simulink model "ModeInputHandle"  (R2018b)
settings: Solver=FixedStepDiscrete  StartTime=0.0  StopTime=10.0  FixedStep=0.01  RelTol=1e-3
undefined symbols (not defined in the file or in its folder): c, CmprtMdHMIReqExt2Tp1, CmprtMdHMIReqExtTp1, CmprtMdHMIReqTp1, d, e, EZESwReq1, f, g, IfVeSMSeStNumConfig, j, KeSMSuButtonLongPressedThrshldTm_Val, KeSMSuFoldType_Val, KeSMSwSeatSMSSeatMdTrigGapTimer_Val, KeSMSwSeatTrigWaitTimer_Val, KeSMSwSRSActiveValidTm_Val, LckUlckActvtFunc1, LstLckFunc1, LugSelectSw1, MdReqTp1, PowerMode1, SeatOccupiedSts1, SRSMode1, StPassCmprtMdCtrl_Md10_VCUConfig_Val, StPassCmprtMdCtrl_Md11_VCUConfig_Val, StPassCmprtMdCtrl_Md12_VCUConfig_Val, StPassCmprtMdCtrl_Md13_VCUConfig_Val, StPassCmprtMdCtrl_Md1_VCUConfig_Val, StPassCmprtMdCtrl_Md27_VCUConfig_Val, StPassCmprtMdCtrl_Md28_VCUConfig_Val, StPassCmprtMdCtrl_Md29_VCUConfig_Val, StPassCmprtMdCtrl_Md2_VCUConfig_Val, StPassCmprtMdCtrl_Md30_VCUConfig_Val, StPassCmprtMdCtrl_Md31_VCUConfig_Val, StPassCmprtMdCtrl_Md32_VCUConfig_Val, StPassCmprtMdCtrl_Md3_VCUConfig_Val, StPassCmprtMdCtrl_Md53_VCUConfig_Val, StPassCmprtMdCtrl_Md56_VCUConfig_Val, StPassCmprtMdCtrl_Md57_VCUConfig_Val, StPassCmprtMdCtrl_Md58_VCUConfig_Val, StPassCmprtMdCtrl_Md61_VCUConfig_Val, StPassCmprtMdCtrl_Md62_VCUConfig_Val, StPassCmprtMdCtrl_Md8_VCUConfig_Val, StPassCmprtMdCtrl_Md9_VCUConfig_Val, StSrv_StMd10_Config_Val, StSrv_StMd11_Config_Val, StSrv_StMd12_Config_Val, StSrv_StMd13_Config_Val, StSrv_StMd1_Config_Val, StSrv_StMd27_Config_Val, StSrv_StMd28_Config_Val, StSrv_StMd29_Config_Val, StSrv_StMd2_Config_Val, StSrv_StMd30_Config_Val, StSrv_StMd31_Config_Val, StSrv_StMd32_Config_Val, StSrv_StMd3_Config_Val, StSrv_StMd8_Config_Val, StSrv_StMd9_Config_Val, VehMovState1
libraries: MSMLib x91
(part 4 of 9)

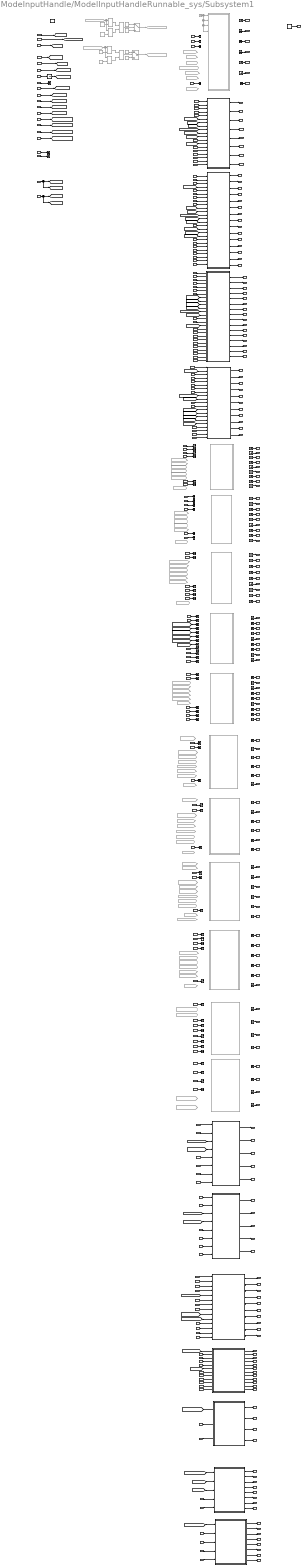
== system ModeInputHandle/ModelInputHandleRunnable_sys/Subsystem1 ==
  note: 2022-02-17:CR202175：修改需求506/548/551/552，新增需求712，完善座椅模式的打断策略。
      | 2023-08-01:新增mode21~26控制接口，REQ_MSM_772/773/774/775//781/784
      | 2024-01-25:对应CT698686:增加KeSMSwSeatTrigWaitTimer，修复休眠情况下无法自动迎宾的问题
  note: //init=[0 1 2 4 3 0 0 0 0 0 0]
  AcsMdExtMdHMI2LRclReq : Inport
  AcsMdExtMdHMI2RRclReq : Inport  Port=2
  AcsMdExtSwLtRclReq : Inport  Port=3
  AcsMdExtSwLtRclReqV : Inport  Port=4
  AcsMdExtSwRtRclReq : Inport  Port=5
  AcsMdExtSwRtRclReqV : Inport  Port=6
  StPassAcsMdExtReq : Inport  Port=7
  SRSCnfmSwReq_67_2 : Inport  Port=8
  StPassCmprtMdHMIReq : Inport  Port=9
  modeAdjustReqDelay : Inport  Port=10
  AcsMdEtrySwRtRclReq : Inport  Port=11
  AcsMdEtrySwRtRclReqV : Inport  Port=12
  AcsEntry2LSwt : Inport  Port=13
  StPassAcsMdEtryReq : Inport  Port=14
  VipMdSwRtRclReq : Inport  Port=15
  VipMdSwRtRclReqV : Inport  Port=16
  Vip2LSwt : Inport  Port=17
  VIPMdHMI2LRclReq : Inport  Port=18
  VIPMdHMI2RRclReq : Inport  Port=19
  StPassVipMdLtReq : Inport  Port=20
  StPassVipMdRtReq : Inport  Port=21
  StSlctSwReq : Inport  Port=22
  StSlctSwReqV : Inport  Port=23
  LugMdSwRclReq : Inport  Port=24
  LugMdSwRclReqV : Inport  Port=25
  StPassLugMdLtReq : Inport  Port=26
  StPassLugMdRtReq : Inport  Port=27
  StPassRcvyMdLtReq : Inport  Port=28
  StPassRcvyMdRtReq : Inport  Port=29
  RcvySwRtReq : Inport  Port=30
  RcvySwRtReqV : Inport  Port=31
  Recovery2LSwt : Inport  Port=32
  RcvyMdHMI2LRclReq : Inport  Port=33
  RcvyMdHMI2RRclReq : Inport  Port=34
  RcvyMdLtAvl : Inport  Port=35
  RcvyMdRtAvl : Inport  Port=36
  ModeSrcTpLt : Inport  Port=37
  KeSMSwSRSActiveValidTm : Inport  Port=38
  KeSMSuButtonLongPressedThrshldTm : Inport  Port=39
  AcsMdExtAvl : Inport  Port=40
  AcsMdEntyAvl : Inport  Port=41
  VipMdLtAvl : Inport  Port=42
  VipMdRtAvl : Inport  Port=43
  LugMdLtAvl : Inport  Port=44
  LugMdRtAvl : Inport  Port=45
  RrRcvyMdSwRclReq : Inport  Port=46
  RrRcvyMdSwRclReqV : Inport  Port=47
  SRSMode : Inport  Port=48
  StPassCmprtMdHMIReqExt : Inport  Port=49
  AcsMdEntyHMI2LRclReq : Inport  Port=50
  AcsMdEntyHMI2RRclReq : Inport  Port=51
  VIPAll2LHMIRclReq : Inport  Port=52
  VIPAll2RHMIRclReq : Inport  Port=53
  Lug2LHMIRclReq : Inport  Port=54
  Lug2RHMIRclReq : Inport  Port=55
  LugAll2LHMIRclReq : Inport  Port=56
  LugAll2RHMIRclReq : Inport  Port=57
  StPassVipAllReq : Inport  Port=58
  StPassLugAllReq : Inport  Port=59
  StPassIntimacyLtMdReq : Inport  Port=60
  StPassIntimacyRtMdReq : Inport  Port=61
  IntimacyLMdHMI2LRclReq : Inport  Port=62
  IntimacyRMdHMI2RRclReq : Inport  Port=63
  IntimacyLMdAvl : Inport  Port=64
  IntimacyRMdAvl : Inport  Port=65
  StPassFamilyMdLtReq : Inport  Port=66
  FamilyMdHMI2LRclReq : Inport  Port=67
  FamilyMdHMI2RRclReq : Inport  Port=68
  FamilyMdLtAvl : Inport  Port=69
  PassFamilyMdRtReq : Inport  Port=70
  FamilyMdRtAvl : Inport  Port=71
  PassLyingMdLtReq : Inport  Port=72
  PassLyingMdRtReq : Inport  Port=73
  LyingMdHMI2LRclReq : Inport  Port=74
  LyingMdHMI2RRclReq : Inport  Port=75
  LyingMdLtAvl : Inport  Port=76
  LyingMdRtAvl : Inport  Port=77
  AcsEntrySwValid : Inport  Port=78
  VipRcvySwValid : Inport  Port=79
  PassLgrstOpenLtMdReq : Inport  Port=80
  PassLgrstCloseLtMdReq : Inport  Port=81
  LgrstOpenLtMdAvl : Inport  Port=82
  LgrstCloseLtMdAvl : Inport  Port=83
  LgrstOpenLtMdHMI2LRclReq : Inport  Port=84
  LgrstCloseLtMdHMI2LRclReq : Inport  Port=85
  PassLgrstOpenRtMdReq : Inport  Port=86
  PassLgrstCloseRtMdReq : Inport  Port=87
  LgrstOpenRtMdAvl : Inport  Port=88
  LgrstCloseRtMdAvl : Inport  Port=89
  LgrstOpenRtMdHMI2RRclReq : Inport  Port=90
  LgrstCloseRtMdHMI2RRclReq : Inport  Port=91
  SRSSlctSwReq : Inport  Port=92
  AcsEntry4s2LAvl : Inport  Port=93
  EZE4SSwReq : Inport  Port=94
  HMIMode21RclReq_2L : Inport  Port=95
  PassAcsEntry4s2LReq : Inport  Port=96
  AcsExit4s2LAvl : Inport  Port=97
  HMIMode22RclReq_2L : Inport  Port=98
  PassAcsExit4s2LReq : Inport  Port=99
  AcsEntry4s2RAvl : Inport  Port=100
  HMIMode23RclReq_2R : Inport  Port=101
  PassAcsEntry4s2RReq : Inport  Port=102
  AcsExit4s2RAvl : Inport  Port=103
  AcsMdExt4SSwRtRclReq : Inport  Port=104
  AcsMdExt4SSwRtRclReqV : Inport  Port=105
  HMIMode24RclReq_2R : Inport  Port=106
  PassAcsExit4s2RReq : Inport  Port=107
  LckUlckActvtFunc : Inport  Port=108
  NotSecRowLeSeaOccStat : Inport  Port=109
  NotSecRowRtSeaOccStat : Inport  Port=110
  SysPwrMd : Inport  Port=111
  SysPwrMdV : Inport  Port=112
  VehMovState : Inport  Port=113
  AcsEntryAll4sFwdAvl : Inport  Port=114
  LstLckFunc : Inport  Port=115
  LstLckChange : Inport  Port=116
  RLDoorAjarSwAct : Inport  Port=117
  RRDoorAjarSwAct : Inport  Port=118
  KeSMSwSeatSMSSeatMdTrigGapTimer : Inport  Port=119
  AcsEntryAll4sBwdAvl : Inport  Port=120
  IfVeSMSeStNumConfig_Val_read : Inport  Port=121
  KeSMSwSeatTrigWaitTimer : Inport  Port=122
  PasReclinerAvl : Inport  Port=123
  PassStFldDnMovSwAct : Inport  Port=124
  PassStFldDnMovSwActV : Inport  Port=125
  PassStFldUpMovSwAct : Inport  Port=126
  PassStFldUpMovSwActV : Inport  Port=127
  StPassPasReclinerEntryReq : Inport  Port=128
  StPassPasReclinerExitReq : Inport  Port=129
  ThdRLtStExpdSwReq : Inport  Port=130
  ThdRLtStExpdSwReqV : Inport  Port=131
  ThdRRtStExpdSwReq : Inport  Port=132
  ThdRRtStExpdSwReqV : Inport  Port=133
  KeSMSuFoldType : Inport  Port=134
  unfold3LAvl : Inport  Port=135
  unfold3RAvl : Inport  Port=136
  VipLtOutMdAvl : Inport  Port=137
  VipRtOutMdAvl : Inport  Port=138
  StPassVIPLtOutReq : Inport  Port=139
  StPassVIPRtOutReq : Inport  Port=140
  StPassVIPAllOutReq : Inport  Port=141
  PasReclinerExitAvl : Inport  Port=142
  StPassCmprtMdHMIReqExt2 : Inport  Port=143
  StPassUnfold3LReq : Inport  Port=144
  Big4SeatAvl : Inport  Port=145
  M61WholeVehMemAvl : Inport  Port=146
  M62WholeVehMemAvl : Inport  Port=147
  StPassCmprtMdCtrl_Md1_VCUConfig : Inport  Port=148
  StPassCmprtMdCtrl_Md10_VCUConfig : Inport  Port=149
  StPassCmprtMdCtrl_Md11_VCUConfig : Inport  Port=150
  StPassCmprtMdCtrl_Md12_VCUConfig : Inport  Port=151
  StPassCmprtMdCtrl_Md13_VCUConfig : Inport  Port=152
  StPassCmprtMdCtrl_Md2_VCUConfig : Inport  Port=153
  StPassCmprtMdCtrl_Md27_VCUConfig : Inport  Port=154
  StPassCmprtMdCtrl_Md28_VCUConfig : Inport  Port=155
  StPassCmprtMdCtrl_Md29_VCUConfig : Inport  Port=156
  StPassCmprtMdCtrl_Md3_VCUConfig : Inport  Port=157
  StPassCmprtMdCtrl_Md30_VCUConfig : Inport  Port=158
  StPassCmprtMdCtrl_Md31_VCUConfig : Inport  Port=159
  StPassCmprtMdCtrl_Md32_VCUConfig : Inport  Port=160
  StPassCmprtMdCtrl_Md53_VCUConfig : Inport  Port=161
  StPassCmprtMdCtrl_Md56_VCUConfig : Inport  Port=162
  StPassCmprtMdCtrl_Md57_VCUConfig : Inport  Port=163
  StPassCmprtMdCtrl_Md58_VCUConfig : Inport  Port=164
  StPassCmprtMdCtrl_Md61_VCUConfig : Inport  Port=165
  StPassCmprtMdCtrl_Md62_VCUConfig : Inport  Port=166
  StPassCmprtMdCtrl_Md8_VCUConfig : Inport  Port=167
  StPassCmprtMdCtrl_Md9_VCUConfig : Inport  Port=168
  StSrv_StMd1_Config : Inport  Port=169
  StSrv_StMd10_Config : Inport  Port=170
  StSrv_StMd11_Config : Inport  Port=171
  StSrv_StMd12_Config : Inport  Port=172
  StSrv_StMd13_Config : Inport  Port=173
  StSrv_StMd2_Config : Inport  Port=174
  StSrv_StMd27_Config : Inport  Port=175
  StSrv_StMd28_Config : Inport  Port=176
  StSrv_StMd29_Config : Inport  Port=177
  StSrv_StMd3_Config : Inport  Port=178
  StSrv_StMd30_Config : Inport  Port=179
  StSrv_StMd31_Config : Inport  Port=180
  StSrv_StMd32_Config : Inport  Port=181
  StSrv_StMd8_Config : Inport  Port=182
  StSrv_StMd9_Config : Inport  Port=183
  AND2 : Logic  Commented=on  Operator=OR  AllPortsSameDT=off  OutDataTypeStr=boolean
  AND3 : Logic  Commented=on  Operator=OR  AllPortsSameDT=off  OutDataTypeStr=boolean
  AcsEntry4s2LMdReq : Subsystem  Commented=on
  "AcsEntry4s2RMdReq " : Subsystem  Commented=on
  AcsEntryAll4sBwdMdReq : Subsystem  Commented=on
  AcsEntryAll4sFwdMdReq : Subsystem  Commented=on
  AcsEntryMdReq : Subsystem
  AcsExit4s2LMdReq : Subsystem  Commented=on
  AcsExit4s2RMdReq : Subsystem  Commented=on
  AcsExtMdReq : Subsystem  Commented=on
  Big4SeatMdReq : Subsystem
  Constant : Constant  Commented=on  Value=IfVeSMSeStNumConfig.SeatNum7Config  OutDataTypeStr=Enum: IfVeSMSeStNumConfig
  Constant1 : Constant  Commented=on  Value=IfVeSMSeStNumConfig.SeatNum6Config  OutDataTypeStr=Enum: IfVeSMSeStNumConfig
  Constant2 : Constant  Commented=on  OutDataTypeStr=boolean
  Constant3 : Constant  Commented=on  Value=0  OutDataTypeStr=boolean
  Constant5 : Constant  Commented=on  Value=IfVeSMSeStNumConfig.SeatNum4Config  OutDataTypeStr=Enum: IfVeSMSeStNumConfig
  Constant6 : Constant  Commented=on  Value=IfVeSMSeStNumConfig.SeatNum4PConfig  OutDataTypeStr=Enum: IfVeSMSeStNumConfig
  Constant7 : Constant  Commented=on  OutDataTypeStr=boolean
  Constant8 : Constant  Commented=on  Value=0  OutDataTypeStr=boolean
  Data Store Memory : DataStoreMemory  DataStoreName=MdSWIntSrc_Val  ReadBeforeWriteMsg=warning  WriteAfterWriteMsg=warning  WriteAfterReadMsg=warning  ShowAdditionalParam=off  OutDataTypeStr=uint16
  Data Store Read : DataStoreRead  DataStoreName=MdSWIntSrc_Val
  Equal{,1..3} (4 alike) : RelationalOperator  Commented=on  Operator===  OutDataTypeStr=boolean  RndMeth=Simplest
  "ExVIPMdReq " : Subsystem
  FamilyMdReq : Subsystem  Commented=on
  From100 : From  Commented=on  GotoTag=NotSecRowRtSeaOccStat
  From{25,38,75,95,101} (5 alike) : From  Commented=on  GotoTag=buttonLongPressedThrshhldTm
  From102 : From  Commented=on  GotoTag=NotSecRowLeSeaOccStat
  From103 : From  Commented=on  GotoTag=NotSecRowRtSeaOccStat
  From105 : From  Commented=on  GotoTag=IfVeSMSeStNumConfig
  From106 : From  Commented=on  GotoTag=IfVeSMSeStNumConfig
  From107 : From  Commented=on  GotoTag=AcsEntry4s2RMdConfig
  From{20,35,61,68,84,91..92} (7 alike) : From  Commented=on  GotoTag=PassCmprtMdHMIReqExt
  From{5,21,40,52,57,62,85,90,98} (9 alike) : From  Commented=on  GotoTag=modeAdjustReqDelay
  From{22,36,53,58,63,69,86,93,230} (9 alike) : From  Commented=on  GotoTag=SRSSlctSwReq
  From{23,37,54,59,65,74,87,94,229} (9 alike) : From  Commented=on  GotoTag=SRSCnfmSwReq
  From{24,41,55,60,66,82,88,96,233} (9 alike) : From  Commented=on  GotoTag=SRSActiveValidTm
  From{26,30,42,71..73,83,89,97} (9 alike) : From  Commented=on  GotoTag=SRSMode
  From{27,46,56,64} (4 alike) : From  Commented=on  GotoTag=passCmprtMdHMIReq
  From28 : From  Commented=on  GotoTag=EZE4SSwReq
  From29 : From  Commented=on  GotoTag=EZE4SSwReq
  From45 : From  Commented=on  GotoTag=AcsMdEtrySwRtRclReq
  From67 : From  Commented=on  GotoTag=AcsMdEtrySwRtRclReqV
  From99 : From  Commented=on  GotoTag=NotSecRowLeSeaOccStat
  Goto122 : Goto  Commented=on  GotoTag=AcsEntry4s2RMdConfig
  Goto69 : Goto  Commented=on  GotoTag=AcsMdEtryConfig
  Ground{,1,3..84} (84 alike) : Ground
  Ground2 : Ground  Commented=on
  IntimacyReq : Subsystem  Commented=on
  LgrstLtMdReq : Subsystem  Commented=on
  LgrstRtMdReq : Subsystem  Commented=on
  LugMdReq : Subsystem
  LyingMdReq : Subsystem  Commented=on
  PasReclinerEntryMdReq : Subsystem
  PasReclinerExitMdReq : Subsystem
  RecoveryMdReq : Subsystem
  Switch : Switch  Commented=on  Criteria=u2 > Threshold
  Switch1 : Switch  Commented=on  Criteria=u2 > Threshold
  Terminator2 : Terminator
  Terminator_{1..68} (68 alike) : Terminator
  UnfoldMdReq : Subsystem
  Unit Delay : UnitDelay  InitialCondition=f  SampleTime=-1
  VIPOutMdReq : Subsystem
  VipMdReq : Subsystem
  WholeVehMem : Subsystem
  acsExtMdReq : Outport
  acsExtMdSrcTp : Outport  Port=2
  SwAcsExtLIntCnt : Outport  Port=3
  SRSAcsExtIntCnt : Outport  Port=4
  acsExtSoftInt : Outport  Port=5
  acsEntyMdReq : Outport  Port=6
  acsEntyMdSrcTp : Outport  Port=7
  SwAcsEntyLIntCnt : Outport  Port=8
  acsEntySoftInt : Outport  Port=9
  SRSAcsEntyIntCnt : Outport  Port=10
  LtVipMdReq : Outport  Port=11
  RtVipMdReq : Outport  Port=12
  AllVipMdReq : Outport  Port=13
  SwLfVipIntCnt : Outport  Port=14
  SwRtVipIntCnt : Outport  Port=15
  SRSAllVipIntCnt : Outport  Port=16
  LtVipSoftInt : Outport  Port=17
  RtVipSoftInt : Outport  Port=18
  LtVipSrcReqTp : Outport  Port=19
  RtVipSrcReqTp : Outport  Port=20
  LtLugMdReq : Outport  Port=21
  RtLugMdReq : Outport  Port=22
  AllLugMdReq : Outport  Port=23
  LtLugSrcReqTp : Outport  Port=24
  RtLugSrcReqTp : Outport  Port=25
  AllLugSrcReqTp : Outport  Port=26
  SwLtLugIntCnt : Outport  Port=27
  SwRtLugIntCnt : Outport  Port=28
  SwAllLugIntCnt : Outport  Port=29
  SRSAllLugIntCnt : Outport  Port=30
  LtLugSoftInt : Outport  Port=31
  RtLugSoftInt : Outport  Port=32
  AllLugSoftInt : Outport  Port=33
  LtRcvyMdReq : Outport  Port=34
  RtRcvyMdReq : Outport  Port=35
  LtRcvySrcReqTp : Outport  Port=36
  RtRcvySrcReqTp : Outport  Port=37
  SwLtRcvyIntCnt : Outport  Port=38
  SwRtRcvyIntCnt : Outport  Port=39
  LtRcvySoftInt : Outport  Port=40
  RtRcvySoftInt : Outport  Port=41
  AllVipSrcReqTp : Outport  Port=42
  AllVipSoftInt : Outport  Port=43
  SRSLfVipIntCnt : Outport  Port=44
  SRSRtVipIntCnt : Outport  Port=45
  SRSLfLugIntCnt : Outport  Port=46
  SRSRtLugIntCnt : Outport  Port=47
  SRSRtRcvyIntCnt : Outport  Port=48
  SRSLtRcvyIntCnt : Outport  Port=49
  SRSIntimacyLtIntCnt : Outport  Port=50
  IntimacyLtMdReq : Outport  Port=51
  IntimacyLtSoftInt : Outport  Port=52
  IntimacyLtMdSrcTp : Outport  Port=53
  SRSIntimacyRtIntCnt : Outport  Port=54
  IntimacyRtMdReq : Outport  Port=55
  IntimacyRtSoftInt : Outport  Port=56
  IntimacyRtMdSrcTp : Outport  Port=57
  SRSFamilyLtIntCnt : Outport  Port=58
  FamilyMdLtReq : Outport  Port=59
  FamilyLtSoftInt : Outport  Port=60
  FamilyLtSrcReqTp : Outport  Port=61
  SRSFamilyRtIntCnt : Outport  Port=62
  FamilyMdRtReq : Outport  Port=63
  FamilyRtSoftInt : Outport  Port=64
  FamilyRtSrcReqTp : Outport  Port=65
  SRSLtLyingIntCnt : Outport  Port=66
  SRSRtLyingIntCnt : Outport  Port=67
  LtLyingMdReq : Outport  Port=68
  LtLyingSoftInt : Outport  Port=69
  LtLyingSrcReqTp : Outport  Port=70
  RtLyingMdReq : Outport  Port=71
  RtLyingSoftInt : Outport  Port=72
  RtLyingSrcReqTp : Outport  Port=73
  SRSLgrstOpenLtIntCnt : Outport  Port=74
  SRSLgrstCloseLtIntCnt : Outport  Port=75
  LgrstOpenLtMdReq : Outport  Port=76
  LgrstOpenLtSoftInt : Outport  Port=77
  LgrstOpenLtSrcReqTp : Outport  Port=78
  LgrstCloseLtMdReq : Outport  Port=79
  LgrstCloseLtSoftInt : Outport  Port=80
  LgrstCloseLtSrcReqTp : Outport  Port=81
  SRSLgrstOpenRtIntCnt : Outport  Port=82
  SRSLgrstCloseRtIntCnt : Outport  Port=83
  LgrstOpenRtMdReq : Outport  Port=84
  LgrstOpenRtSoftInt : Outport  Port=85
  LgrstOpenRtSrcReqTp : Outport  Port=86
  LgrstCloseRtMdReq : Outport  Port=87
  LgrstCloseRtSoftInt : Outport  Port=88
  LgrstCloseRtSrcReqTp : Outport  Port=89
  SwAcsExtRIntCnt : Outport  Port=90
  SwAcsEntyRIntCnt : Outport  Port=91
  SwAcsEntyBIntCnt : Outport  Port=92
      settings: EnsureOutportIsVirtual=on
  acsMdExtNotf1ChimeEventStat : Outport  Port=93
  acsMdEntryNotf1ChimeEventStat : Outport  Port=94
  VipMdNotf1ChimeEventStat : Outport  Port=95
  LugMdNotf1ChimeEventStat : Outport  Port=96
  RcvyMdNotf1ChimeEventStat : Outport  Port=97
  IntimacyMdNotf1ChimeEventStat : Outport  Port=98
  FamilyMdNotf1ChimeEventStat : Outport  Port=99
  LyingMdNotf1ChimeEventStat : Outport  Port=100
  LgrstLtMdNotf1ChimeEventStat : Outport  Port=101
  LgrstRtMdNotf1ChimeEventStat : Outport  Port=102
  MdSWIntSrc : Outport  Port=103
  acsEntry4s2LReq : Outport  Port=104
  acsEntry4s2LSoftInt : Outport  Port=105
  acsEntry4s2LSrcTp : Outport  Port=106
  SwAcsEntry4s2LIntCnt : Outport  Port=107
  AcsEntry4s2LNotf1ChimeEventStat : Outport  Port=108
  SRSAcsEntry4s2LIntCnt : Outport  Port=109
  acsExit4s2LReq : Outport  Port=110
  acsExit4s2LSoftInt : Outport  Port=111
  SwAcsExit4s2LIntCnt : Outport  Port=112
  AcsExit4s2LNotf1ChimeEventStat : Outport  Port=113
  acsExit4s2LSrcTp : Outport  Port=114
  SRSAcsExit4s2LIntCnt : Outport  Port=115
  SwAcsEntry4s2RIntCnt : Outport  Port=116
  acsEntry4s2RReq : Outport  Port=117
  acsEntry4s2RSoftInt : Outport  Port=118
  AcsEntry4s2RNotf1ChimeEventStat : Outport  Port=119
  acsEntry4s2RSrcTp : Outport  Port=120
  SRSAcsEntry4s2RIntCnt : Outport  Port=121
  acsExit4s2RSoftInt : Outport  Port=122
  acsExit4s2RReq : Outport  Port=123
  AcsExit4s2RNotf1ChimeEventStat : Outport  Port=124
  SwAcsExit4s2RIntCnt : Outport  Port=125
  acsExit4s2RSrcTp : Outport  Port=126
  SRSAcsExit4s2RIntCnt : Outport  Port=127
  acsEntryAll4sFwdReq : Outport  Port=128
  acsEntryAll4sFwdSoftInt : Outport  Port=129
  AcsEntryAll4sFwdNotf1ChimeEventStat : Outport  Port=130
  acsEntryAll4sBwdReq : Outport  Port=131
  acsEntryAll4sBwdSoftInt : Outport  Port=132
  acsEntryAll4sBwdNotf1ChimeEventStat : Outport  Port=133
  acsEntryAll4sFwdReqSig : Outport  Port=134
  acsEntryAll4sBwdReqSig : Outport  Port=135
  SwPasReclinerEntryIntCnt : Outport  Port=136
  PasReclinerEntryReq : Outport  Port=137
  PasReclinerEntrySrcReqTp : Outport  Port=138
  PasReclinerEntrySoftInt : Outport  Port=139
  PasReclinerEntryNotf1ChimeEventStat : Outport  Port=140
  SwPasReclinerExitIntCnt : Outport  Port=141
  PasReclinerExitReq : Outport  Port=142
  PasReclinerExitSrcReqTp : Outport  Port=143
  PasReclinerExitSoftInt : Outport  Port=144
  PasReclinerExitNotf1ChimeEventStat : Outport  Port=145
  SwUnfold3LIntCnt : Outport  Port=146
  SwUnfold3RIntCnt : Outport  Port=147
  Unfold3LReq : Outport  Port=148
  Unfold3LsrcReqTp : Outport  Port=149
  Unfold3LNotf1ChimeEventStat : Outport  Port=150
  Unfold3RReq : Outport  Port=151
  Unfold3RsrcReqTp : Outport  Port=152
  Unfold3RNotf1ChimeEventStat : Outport  Port=153
  VIPLtOutReq : Outport  Port=154
  VIPLtOutsrcReqTp : Outport  Port=155
  VIPLtOutSoftInt : Outport  Port=156
  VIPLtOutNotf1ChimeEventStat : Outport  Port=157
  VIPRtOutReq : Outport  Port=158
  VIPRtOutsrcReqTp : Outport  Port=159
  VIPRtOutSoftInt : Outport  Port=160
  VIPRtOutNotf1ChimeEventStat : Outport  Port=161
  VIPAllOutReq : Outport  Port=162
  VIPAllOutsrcReqTp : Outport  Port=163
  VIPAllOutSoftInt : Outport  Port=164
  VIPAllOutNotf1ChimeEventStat : Outport  Port=165
  Big4SeatNotf1ChimeEventStat : Outport  Port=166
  Big4SeatReq : Outport  Port=167
  Big4SeatSoftInt : Outport  Port=168
  Big4SeatsrcReqTp : Outport  Port=169
  Unfold3LSoftInt : Outport  Port=170
  Unfold3RSoftInt : Outport  Port=171
  "ExVIPRReq " : Outport  Port=172
  ExVIPRsrcReqTp : Outport  Port=173
  ExVIPRSoftInt : Outport  Port=174
  ExVIPRNotf1ChimeEventStat : Outport  Port=175
  ExVIPROutReq : Outport  Port=176
  ExVIPROutsrcReqTp : Outport  Port=177
  ExVIPROutSoftInt : Outport  Port=178
  ExVIPROutNotf1ChimeEventStat : Outport  Port=179
  WholeVehMem1Req : Outport  Port=180
  WholeVehMem1Notf1ChimeEventStat : Outport  Port=181
  WholeVehMem1SoftInt : Outport  Port=182
  WholeVehMem1srcReqTp : Outport  Port=183
  WholeVehMem2Notf1ChimeEventStat : Outport  Port=184
  WholeVehMem2Req : Outport  Port=185
  WholeVehMem2SoftInt : Outport  Port=186
  WholeVehMem2srcReqTp : Outport  Port=187
  wires:
  RecoveryMdReq/2(RtRcvyMdReq) -> RtRcvyMdReq/1
  SRSMode/1 -> [SRSMode]
  StPassCmprtMdHMIReqExt/1 -> [PassCmprtMdHMIReqExt]
  StPassCmprtMdHMIReq/1 -> [passCmprtMdHMIReq]
  [SRSMode] -> LugMdReq/16(SRSMode)
  SRSSlctSwReq/1 -> [SRSSlctSwReq]
  AcsEntryMdReq/8(SwAcsEntyBIntCnt) -> SwAcsEntyBIntCnt/1
  RcvyMdRtAvl/1 -> RecoveryMdReq/12(RcvyMdRtAvl)
  [SRSMode] -> AcsEntryMdReq/13(SRSMode)
  [SRSActiveValidTm] -> AcsEntryMdReq/11(SRSActiveValidTm)
  AcsEntryMdReq/2(srcReqTp) -> acsEntyMdSrcTp/1
  Lug2RHMIRclReq/1 -> LugMdReq/18(HMI2RRclReq)
  [SRSCnfmSwReq] -> VipMdReq/11(SRSCnfmSwReq)
  VipMdReq/9("LtVipSrcReqTp ") -> LtVipSrcReqTp/1
  VipMdSwRtRclReqV/1 -> VipMdReq/2(SwRtRclReqV)
  LugMdReq/15(SRSLfLugIntCnt) -> SRSLfLugIntCnt/1
  VipMdLtAvl/1 -> VipMdReq/15(VipMdLtAvl)
  [modeAdjustReqDelay] -> AcsEntryMdReq/10(curMode)
  StPassVipAllReq/1 -> VipMdReq/9(PassVipAllReq)
  [SRSActiveValidTm] -> VipMdReq/14(SRSActiveValidTm)
  StSlctSwReqV/1 -> LugMdReq/2(SlctSwReqV)
  SRSCnfmSwReq_67_2/1 -> [SRSCnfmSwReq]
  [SRSCnfmSwReq] -> LugMdReq/10(SRSCnfmSwReq)
  RcvyMdLtAvl/1 -> RecoveryMdReq/11(RcvyMdLtAvl)
  LugAll2LHMIRclReq/1 -> LugMdReq/19(LugAll2LHMIRclReq)
  modeAdjustReqDelay/1 -> Unit Delay/1
  LugMdReq/5(RtLugSrcReqTp) -> RtLugSrcReqTp/1
  [SRSSlctSwReq] -> LugMdReq/9(SRSSlctSwReq)
  RecoveryMdReq/10(SRSRtRcvyIntCnt) -> SRSRtRcvyIntCnt/1
  Lug2LHMIRclReq/1 -> LugMdReq/17(HMI2LRclReq)
  VipMdReq/6(SRSAllVipIntCnt) -> SRSAllVipIntCnt/1
  StPassVipMdLtReq/1 -> VipMdReq/7(PassVipMdLtReq)
  StPassAcsMdEtryReq/1 -> AcsEntryMdReq/5(PassAcsMdEtryReq)
  LugMdReq/4(LtLugSrcReqTp) -> LtLugSrcReqTp/1
  StPassVipMdRtReq/1 -> VipMdReq/8(PassVipMdRtReq)
  LugMdReq/7(SwLtLugIntCnt) -> SwLtLugIntCnt/1
  VIPMdHMI2RRclReq/1 -> VipMdReq/6(HMI2RRclReq)
  VipMdSwRtRclReq/1 -> VipMdReq/1(SwRtRclReq)
  KeSMSuButtonLongPressedThrshldTm/1 -> [buttonLongPressedThrshhldTm]
  [SRSCnfmSwReq] -> AcsEntryMdReq/8(SRSCnfmSwReq)
  [modeAdjustReqDelay] -> LugMdReq/13(curMode)
  [buttonLongPressedThrshhldTm] -> AcsEntryMdReq/9(buttonLongPressedThrshhldTm)
  [VipRcvySwValid] -> VipMdReq/4(VipSwValid)
  StPassLugAllReq/1 -> LugMdReq/7(PassLugAllReq)
  RrRcvyMdSwRclReqV/1 -> AcsEntryMdReq/15(RrRcvyMdSwRclReqV)
  [SRSSlctSwReq] -> RecoveryMdReq/14(SRSSlctSwReq)
  AcsEntryMdReq/4(acsEntySoftInt) -> acsEntySoftInt/1
  RecoveryMdReq/5(Sw2LRcvyIntCnt) -> SwLtRcvyIntCnt/1
  RcvyMdHMI2RRclReq/1 -> RecoveryMdReq/8(RcvyMdHMI2RRclReq)
  VipMdReq/14(SRSLfVipIntCnt) -> SRSLfVipIntCnt/1
  [buttonLongPressedThrshhldTm] -> LugMdReq/12(buttonLongPressedThrshhldTm)
  [SRSActiveValidTm] -> RecoveryMdReq/16(SRSActiveValidTm)
  StPassRcvyMdLtReq/1 -> RecoveryMdReq/5(PassRcvyMdLtReq)
  VipMdReq/15(SRSRtVipIntCnt) -> SRSRtVipIntCnt/1
  [SRSMode] -> VipMdReq/17(SRSMode)
  LugMdReq/13(RtLugSoftInt) -> RtLugSoftInt/1
  VipMdReq/8(RtVipSoftInt) -> RtVipSoftInt/1
  LugMdSwRclReqV/1 -> LugMdReq/4(SwConfmReqV)
  StPassRcvyMdRtReq/1 -> RecoveryMdReq/6(PassRcvyMdRtReq)
  AcsEntryMdReq/5(SRSAcsEntyIntCnt) -> SRSAcsEntyIntCnt/1
  [VipRcvySwValid] -> RecoveryMdReq/2(RcvySwValid)
  RecoveryMdReq/9(RtRcvySoftInt) -> RtRcvySoftInt/1
  LugMdReq/11(Notf1ChimeEventStat) -> LugMdNotf1ChimeEventStat/1
  RecoveryMdReq/3(LtRcvySrcReqTp) -> LtRcvySrcReqTp/1
  [passCmprtMdHMIReq] -> RecoveryMdReq/13(passCmprtMdHMIReq)
  [passCmprtMdHMIReq] -> LugMdReq/8(passCmprtMdHMIReq)
  VipRcvySwValid/1 -> [VipRcvySwValid]
  VipMdReq/1(LtVipMdReq) -> LtVipMdReq/1
  [buttonLongPressedThrshhldTm] -> VipMdReq/12(buttonLongPressedThrshhldTm)
  Unit Delay/1 -> [modeAdjustReqDelay]
  [SRSSlctSwReq] -> VipMdReq/10(SRSSlctSwReq)
  LugMdReq/9(SwAllLugIntCnt) -> SwAllLugIntCnt/1
  VipMdReq/4(SwLfVipIntCnt) -> SwLfVipIntCnt/1
  RecoveryMdReq/6(SwRtRcvyIntCnt) -> SwRtRcvyIntCnt/1
  [passCmprtMdHMIReq] -> VipMdReq/18(passCmprtMdHMIReq)
  RcvyMdHMI2LRclReq/1 -> RecoveryMdReq/7(RcvyMdHMI2LRclReq)
  [SRSSlctSwReq] -> AcsEntryMdReq/7(SRSSlctSwReq)
  RecoveryMdReq/11(SRSLtRcvyIntCnt) -> SRSLtRcvyIntCnt/1
  [SRSActiveValidTm] -> LugMdReq/11(SRSActiveValidTm)
  AcsEntryMdReq/3("SwAcsEntyLIntCnt ") -> SwAcsEntyLIntCnt/1
  VipMdReq/11(Notf1ChimeEventStat) -> VipMdNotf1ChimeEventStat/1
  LugMdReq/14(AllLugSoftInt) -> AllLugSoftInt/1
  StPassLugMdLtReq/1 -> LugMdReq/5(PassLugMdLtReq)
  LugAll2RHMIRclReq/1 -> LugMdReq/20(LugAll2RHMIRclReq)
  Recovery2LSwt/1 -> RecoveryMdReq/1(Recovery2LSwt)
  RecoveryMdReq/4(RtRcvySrcReqTp) -> RtRcvySrcReqTp/1
  VIPMdHMI2LRclReq/1 -> VipMdReq/5(HMI2LRclReq)
  VipMdReq/2(RtVipMdReq) -> RtVipMdReq/1
  VipMdReq/10("RtVipSrcReqTp ") -> RtVipSrcReqTp/1
  VIPAll2RHMIRclReq/1 -> VipMdReq/20(VipAll2RHMIRclReq)
  VipMdReq/13(AllVipSoftInt) -> AllVipSoftInt/1
  LugMdReq/3(AllLugMdReq) -> AllLugMdReq/1
  LugMdRtAvl/1 -> LugMdReq/15(LugMdRtAvl)
  LugMdReq/2(RtLugMdReq) -> RtLugMdReq/1
  ModeSrcTpLt/1 -> Terminator2/1
  VipMdReq/5(SwRtVipIntCnt) -> SwRtVipIntCnt/1
  Vip2LSwt/1 -> VipMdReq/3(SwLfRclReq)
  LugMdLtAvl/1 -> LugMdReq/14(LugMdLtAvl)
  VipMdReq/12(AllVipSrcReqTp) -> AllVipSrcReqTp/1
  RecoveryMdReq/1(LtRcvyMdReq) -> LtRcvyMdReq/1
  RrRcvyMdSwRclReq/1 -> AcsEntryMdReq/14(RrRcvyMdSwRclReq)
  VipMdReq/7(LtVipSoftInt) -> LtVipSoftInt/1
  [modeAdjustReqDelay] -> VipMdReq/13(curMode)
  RecoveryMdReq/8(LtRcvySoftInt) -> LtRcvySoftInt/1
  KeSMSwSRSActiveValidTm/1 -> [SRSActiveValidTm]
  AcsEntryMdReq/1(acsEntyMdReq) -> acsEntyMdReq/1
  LugMdReq/8(SwRtLugIntCnt) -> SwRtLugIntCnt/1
  RecoveryMdReq/7(Notf1ChimeEventStat) -> RcvyMdNotf1ChimeEventStat/1
  [buttonLongPressedThrshhldTm] -> RecoveryMdReq/9(buttonLongPressedThrshhldTm)
  LugMdReq/16(SRSRtLugIntCnt) -> SRSRtLugIntCnt/1
  LugMdReq/10(SRSAllLugIntCnt) -> SRSAllLugIntCnt/1
  [SRSMode] -> RecoveryMdReq/17(SRSMode)
  RcvySwRtReq/1 -> RecoveryMdReq/3(RcvySwRtReq)
  StPassLugMdRtReq/1 -> LugMdReq/6(PassLugMdRtReq)
  RcvySwRtReqV/1 -> RecoveryMdReq/4(RcvySwRtReqV)
  LugMdReq/1(LtLugMdReq) -> LtLugMdReq/1
  LugMdReq/6(AllLugSrcReqTp) -> AllLugSrcReqTp/1
  VipMdReq/3(AllVipMdReq) -> AllVipMdReq/1
  [modeAdjustReqDelay] -> RecoveryMdReq/10(curMode)
  StSlctSwReq/1 -> LugMdReq/1(SlctSwReq)
  LugMdReq/12(LtLugSoftInt) -> LtLugSoftInt/1
  AcsEntryMdReq/6(Notf1ChimeEventStat) -> acsMdEntryNotf1ChimeEventStat/1
  [passCmprtMdHMIReq] -> AcsEntryMdReq/6(passCmprtMdHMIReq)
  AcsEntryMdReq/7(SwAcsEntyRIntCnt) -> SwAcsEntyRIntCnt/1
  LugMdSwRclReq/1 -> LugMdReq/3(SwConfmReq)
  VIPAll2LHMIRclReq/1 -> VipMdReq/19(VipAll2LHMIRclReq)
  [SRSCnfmSwReq] -> RecoveryMdReq/15(SRSCnfmSwReq)
  Data Store Read/1 -> MdSWIntSrc/1
  EZE4SSwReq/1 -> [EZE4SSwReq]
  AcsMdEtrySwRtRclReq/1 -> [AcsMdEtrySwRtRclReq]
  AcsMdEtrySwRtRclReqV/1 -> [AcsMdEtrySwRtRclReqV]
  NotSecRowLeSeaOccStat/1 -> [NotSecRowLeSeaOccStat]
  NotSecRowRtSeaOccStat/1 -> [NotSecRowRtSeaOccStat]
  IfVeSMSeStNumConfig_Val_read/1 -> [IfVeSMSeStNumConfig]
  AND3/1 -> Switch1/2
  Equal1/1 -> AND2/2
  Constant5/1 -> Equal2/2
  Switch/1 -> Goto69/1
  Switch1/1 -> Goto122/1
  Equal3/1 -> AND3/2
  Constant6/1 -> Equal3/2
  Constant2/1 -> Switch/1
  Constant7/1 -> Switch1/1
  Constant3/1 -> Switch/3
  Equal2/1 -> AND3/1
  AND2/1 -> Switch/2
  Constant8/1 -> Switch1/3
  Constant1/1 -> Equal1/2
  Equal/1 -> AND2/1
  From105/1 -> Equal1/1, Equal/1
  Constant/1 -> Equal/2
  From106/1 -> Equal3/1, Equal2/1
  PassStFldDnMovSwAct/1 -> PasReclinerEntryMdReq/1(PassStFldDnMovSwAct)
  PassStFldDnMovSwActV/1 -> PasReclinerEntryMdReq/2(PassStFldDnMovSwActV)
  PasReclinerEntryMdReq/1(SwPasReclinerEntryIntCnt) -> SwPasReclinerEntryIntCnt/1
  [buttonLongPressedThrshhldTm] -> PasReclinerEntryMdReq/3(buttonLongPressedThrshhldTm)
  StPassPasReclinerEntryReq/1 -> PasReclinerEntryMdReq/5(PassPasReclinerEntryReq)
  PasReclinerEntryMdReq/2(PasReclinerEntryReq) -> PasReclinerEntryReq/1
  PasReclinerEntryMdReq/3(srcReqTp) -> PasReclinerEntrySrcReqTp/1
  PasReclinerEntryMdReq/4(PasReclinerEntrySoftInt) -> PasReclinerEntrySoftInt/1
  PasReclinerEntryMdReq/5(Notf1ChimeEventStat) -> PasReclinerEntryNotf1ChimeEventStat/1
  [buttonLongPressedThrshhldTm] -> PasReclinerExitMdReq/3(buttonLongPressedThrshhldTm)
  [PassCmprtMdHMIReqExt] -> PasReclinerExitMdReq/4(PassCmprtMdHMIReqExt)
  PassStFldUpMovSwAct/1 -> PasReclinerExitMdReq/1(PassStFldUpMovSwAct)
  PassStFldUpMovSwActV/1 -> PasReclinerExitMdReq/2(PassStFldUpMovSwActV)
  StPassPasReclinerExitReq/1 -> PasReclinerExitMdReq/5(PassPasReclinerExitReq)
  PasReclinerExitMdReq/1(SwPasReclinerExitIntCnt) -> SwPasReclinerExitIntCnt/1
  PasReclinerExitMdReq/2(PasReclinerExitReq) -> PasReclinerExitReq/1
  PasReclinerExitMdReq/3(srcReqTp) -> PasReclinerExitSrcReqTp/1
  PasReclinerExitMdReq/4(PasReclinerExitSoftInt) -> PasReclinerExitSoftInt/1
  PasReclinerExitMdReq/5(Notf1ChimeEventStat) -> PasReclinerExitNotf1ChimeEventStat/1
  UnfoldMdReq/1(SwUnfold3LIntCnt) -> SwUnfold3LIntCnt/1
  [buttonLongPressedThrshhldTm] -> UnfoldMdReq/5(buttonLongPressedThrshhldTm)
  ThdRLtStExpdSwReq/1 -> UnfoldMdReq/1(ThdRLtStExpdSwReq)
  ThdRLtStExpdSwReqV/1 -> UnfoldMdReq/2(ThdRLtStExpdSwReqV)
  ThdRRtStExpdSwReqV/1 -> UnfoldMdReq/4(ThdRRtStExpdSwReqV)
  ThdRRtStExpdSwReq/1 -> UnfoldMdReq/3(ThdRRtStExpdSwReq)
  KeSMSuFoldType/1 -> UnfoldMdReq/6(KeSMSuFoldType)
  unfold3LAvl/1 -> UnfoldMdReq/7(unfold3LAvl)
  unfold3RAvl/1 -> UnfoldMdReq/8(unfold3RAvl)
  UnfoldMdReq/2(SwUnfold3RIntCnt) -> SwUnfold3RIntCnt/1
  UnfoldMdReq/3(Unfold3LReq) -> Unfold3LReq/1
  UnfoldMdReq/4(Unfold3LsrcReqTp) -> Unfold3LsrcReqTp/1
  UnfoldMdReq/5(Unfold3LNotf1ChimeEventStat) -> Unfold3LNotf1ChimeEventStat/1
  UnfoldMdReq/6(Unfold3RReq) -> Unfold3RReq/1
  UnfoldMdReq/7(Unfold3RsrcReqTp) -> Unfold3RsrcReqTp/1
  UnfoldMdReq/8(Unfold3RNotf1ChimeEventStat) -> Unfold3RNotf1ChimeEventStat/1
  StPassVIPLtOutReq/1 -> VIPOutMdReq/2(PassVIPLtOutReq)
  StPassVIPRtOutReq/1 -> VIPOutMdReq/3(PassVIPRtOutReq)
  StPassVIPAllOutReq/1 -> VIPOutMdReq/4(PassVIPAllOutReq)
  VipLtOutMdAvl/1 -> VIPOutMdReq/5(VipLtOutMdAvl)
  VIPOutMdReq/1(VIPLtOutReq) -> VIPLtOutReq/1
  VIPOutMdReq/2(VIPLtOutsrcReqTp) -> VIPLtOutsrcReqTp/1
  VIPOutMdReq/3(VIPLtOutSoftInt) -> VIPLtOutSoftInt/1
  VIPOutMdReq/4(VIPLtOutNotf1ChimeEventStat) -> VIPLtOutNotf1ChimeEventStat/1
  VIPOutMdReq/5(VIPRtOutReq) -> VIPRtOutReq/1
  VIPOutMdReq/6(VIPRtOutsrcReqTp) -> VIPRtOutsrcReqTp/1
  VIPOutMdReq/7(VIPRtOutSoftInt) -> VIPRtOutSoftInt/1
  VIPOutMdReq/8(VIPRtOutNotf1ChimeEventStat) -> VIPRtOutNotf1ChimeEventStat/1
  VIPOutMdReq/9(VIPAllOutReq) -> VIPAllOutReq/1
  VIPOutMdReq/10(VIPAllOutsrcReqTp) -> VIPAllOutsrcReqTp/1
  VIPOutMdReq/11(VIPAllOutSoftInt) -> VIPAllOutSoftInt/1
  VIPOutMdReq/12(VIPAllOutNotf1ChimeEventStat) -> VIPAllOutNotf1ChimeEventStat/1
  Ground2/1 -> AcsExtMdReq/4(SwLtRclReqV), AcsExtMdReq/3(SwLtRclReq), AcsExtMdReq/2(SwRtRclReqV), AcsExtMdReq/1(SwRtRclReq)
  AcsEntry2LSwt/1 -> Terminator_59/1
  AcsEntrySwValid/1 -> Terminator_1/1
  AcsMdExtSwLtRclReq/1 -> AcsEntryMdReq/1(AcsMdExtSwLtRclReq)
  AcsMdExtSwLtRclReqV/1 -> AcsEntryMdReq/2(AcsMdExtSwLtRclReqV)
  AcsMdExtSwRtRclReq/1 -> AcsEntryMdReq/3(AcsMdExtSwRtRclReq)
  AcsMdExtSwRtRclReqV/1 -> AcsEntryMdReq/4(AcsMdExtSwRtRclReqV)
  [PassCmprtMdHMIReqExt] -> PasReclinerEntryMdReq/4(PassCmprtMdHMIReqExt)
  [PassCmprtMdHMIReqExt] -> VIPOutMdReq/1(PassCmprtMdHMIReqExt)
  PasReclinerExitAvl/1 -> PasReclinerExitMdReq/6(PasReclinerExitAvl)
  PasReclinerAvl/1 -> PasReclinerEntryMdReq/6(PasReclinerAvl)
  StPassIntimacyLtMdReq/1 -> Terminator_2/1
  StPassIntimacyRtMdReq/1 -> Terminator_3/1
  IntimacyLMdHMI2LRclReq/1 -> Terminator_4/1
  IntimacyRMdHMI2RRclReq/1 -> Terminator_5/1
  IntimacyLMdAvl/1 -> Terminator_6/1
  IntimacyRMdAvl/1 -> Terminator_7/1
  Ground/1 -> SRSIntimacyLtIntCnt/1
  Ground1/1 -> IntimacyLtMdReq/1
  Ground3/1 -> IntimacyLtSoftInt/1
  Ground4/1 -> IntimacyLtMdSrcTp/1
  Ground5/1 -> SRSIntimacyRtIntCnt/1
  Ground6/1 -> IntimacyMdNotf1ChimeEventStat/1
  Ground7/1 -> IntimacyRtMdReq/1
  Ground8/1 -> IntimacyRtSoftInt/1
  Ground9/1 -> IntimacyRtMdSrcTp/1
  StPassFamilyMdLtReq/1 -> Terminator_8/1
  PassFamilyMdRtReq/1 -> Terminator_9/1
  FamilyMdHMI2LRclReq/1 -> Terminator_10/1
  FamilyMdLtAvl/1 -> Terminator_12/1
  FamilyMdRtAvl/1 -> Terminator_13/1
  Ground10/1 -> SRSFamilyLtIntCnt/1
  Ground11/1 -> FamilyMdLtReq/1
  Ground12/1 -> FamilyLtSoftInt/1
  Ground13/1 -> FamilyLtSrcReqTp/1
  Ground14/1 -> SRSFamilyRtIntCnt/1
  Ground15/1 -> FamilyMdRtReq/1
  Ground16/1 -> FamilyRtSoftInt/1
  Ground17/1 -> FamilyRtSrcReqTp/1
  Ground18/1 -> FamilyMdNotf1ChimeEventStat/1
  Ground19/1 -> SRSLtLyingIntCnt/1
  Ground20/1 -> SRSRtLyingIntCnt/1
  Ground21/1 -> LtLyingMdReq/1
  Ground22/1 -> LtLyingSoftInt/1
  Ground23/1 -> LtLyingSrcReqTp/1
  Ground24/1 -> RtLyingMdReq/1
  Ground25/1 -> RtLyingSoftInt/1
  Ground26/1 -> RtLyingSrcReqTp/1
  Ground27/1 -> LyingMdNotf1ChimeEventStat/1
  PassLyingMdLtReq/1 -> Terminator_14/1
  PassLyingMdRtReq/1 -> Terminator_15/1
  LyingMdHMI2LRclReq/1 -> Terminator_16/1
  LyingMdHMI2RRclReq/1 -> Terminator_17/1
  LyingMdLtAvl/1 -> Terminator_18/1
  LyingMdRtAvl/1 -> Terminator_19/1
  Ground28/1 -> SRSLgrstOpenLtIntCnt/1
  Ground29/1 -> SRSLgrstCloseLtIntCnt/1
  Ground30/1 -> LgrstOpenLtMdReq/1
  Ground31/1 -> LgrstOpenLtSoftInt/1
  Ground32/1 -> LgrstOpenLtSrcReqTp/1
  Ground33/1 -> LgrstCloseLtMdReq/1
  Ground34/1 -> LgrstCloseLtSoftInt/1
  Ground35/1 -> LgrstCloseLtSrcReqTp/1
  Ground36/1 -> LgrstLtMdNotf1ChimeEventStat/1
  PassLgrstOpenLtMdReq/1 -> Terminator_20/1
  PassLgrstCloseLtMdReq/1 -> Terminator_21/1
  [PassCmprtMdHMIReqExt] -> Terminator_22/1
  [modeAdjustReqDelay] -> Terminator_23/1
  [SRSSlctSwReq] -> Terminator_24/1
  [SRSCnfmSwReq] -> Terminator_25/1
  [SRSActiveValidTm] -> Terminator_26/1
  [SRSMode] -> Terminator_27/1
  LgrstOpenLtMdAvl/1 -> Terminator_28/1
  LgrstCloseLtMdAvl/1 -> Terminator_29/1
  LgrstOpenLtMdHMI2LRclReq/1 -> Terminator_30/1
  LgrstCloseLtMdHMI2LRclReq/1 -> Terminator_31/1
  Ground37/1 -> SRSLgrstOpenRtIntCnt/1
  Ground38/1 -> SRSLgrstCloseRtIntCnt/1
  Ground39/1 -> LgrstOpenRtMdReq/1
  Ground40/1 -> LgrstOpenRtSoftInt/1
  Ground41/1 -> LgrstOpenRtSrcReqTp/1
  Ground42/1 -> LgrstCloseRtMdReq/1
  Ground43/1 -> LgrstCloseRtSoftInt/1
  Ground44/1 -> LgrstCloseRtSrcReqTp/1
  Ground45/1 -> LgrstRtMdNotf1ChimeEventStat/1
  PassLgrstOpenRtMdReq/1 -> Terminator_32/1
  PassLgrstCloseRtMdReq/1 -> Terminator_33/1
  LgrstOpenRtMdAvl/1 -> Terminator_34/1
  LgrstCloseRtMdAvl/1 -> Terminator_35/1
  LgrstOpenRtMdHMI2RRclReq/1 -> Terminator_36/1
  LgrstCloseRtMdHMI2RRclReq/1 -> Terminator_37/1
  Ground46/1 -> acsEntry4s2LReq/1
  Ground47/1 -> acsEntry4s2LSrcTp/1
  Ground48/1 -> SwAcsEntry4s2LIntCnt/1
  Ground49/1 -> SRSAcsEntry4s2LIntCnt/1
  Ground50/1 -> AcsEntry4s2LNotf1ChimeEventStat/1
  Ground51/1 -> acsEntry4s2LSoftInt/1
  HMIMode21RclReq_2L/1 -> Terminator_38/1
  PassAcsEntry4s2LReq/1 -> Terminator_39/1
  AcsEntry4s2LAvl/1 -> Terminator_40/1
  Ground52/1 -> acsExit4s2LReq/1
  Ground53/1 -> acsExit4s2LSrcTp/1
  Ground54/1 -> SwAcsExit4s2LIntCnt/1
  Ground55/1 -> SRSAcsExit4s2LIntCnt/1
  Ground56/1 -> AcsExit4s2LNotf1ChimeEventStat/1
  Ground57/1 -> acsExit4s2LSoftInt/1
  HMIMode22RclReq_2L/1 -> Terminator_41/1
  PassAcsExit4s2LReq/1 -> Terminator_42/1
  AcsExit4s2LAvl/1 -> Terminator_43/1
  Ground58/1 -> acsEntry4s2RReq/1
  Ground59/1 -> acsEntry4s2RSrcTp/1
  Ground60/1 -> SwAcsEntry4s2RIntCnt/1
  Ground61/1 -> SRSAcsEntry4s2RIntCnt/1
  Ground62/1 -> AcsEntry4s2RNotf1ChimeEventStat/1
  Ground63/1 -> acsEntry4s2RSoftInt/1
  HMIMode23RclReq_2R/1 -> Terminator_44/1
  PassAcsEntry4s2RReq/1 -> Terminator_45/1
  AcsEntry4s2RAvl/1 -> Terminator_46/1
  Ground64/1 -> acsExit4s2RReq/1
  Ground65/1 -> acsExit4s2RSrcTp/1
  Ground66/1 -> SwAcsExit4s2RIntCnt/1
  Ground67/1 -> SRSAcsExit4s2RIntCnt/1
  Ground68/1 -> AcsExit4s2RNotf1ChimeEventStat/1
  Ground69/1 -> acsExit4s2RSoftInt/1
  AcsMdExt4SSwRtRclReq/1 -> Terminator_47/1
  AcsMdExt4SSwRtRclReqV/1 -> Terminator_48/1
  HMIMode24RclReq_2R/1 -> Terminator_49/1
  PassAcsExit4s2RReq/1 -> Terminator_50/1
  AcsExit4s2RAvl/1 -> Terminator_51/1
  Ground70/1 -> acsEntryAll4sFwdReq/1
  Ground71/1 -> acsEntryAll4sFwdSoftInt/1
  Ground72/1 -> AcsEntryAll4sFwdNotf1ChimeEventStat/1
  Ground73/1 -> acsEntryAll4sFwdReqSig/1
  LckUlckActvtFunc/1 -> Terminator_52/1
  SysPwrMd/1 -> Terminator_53/1
  SysPwrMdV/1 -> Terminator_54/1
  VehMovState/1 -> Terminator_55/1
  AcsEntryAll4sFwdAvl/1 -> Terminator_56/1
  LstLckFunc/1 -> Terminator_57/1
  LstLckChange/1 -> Terminator_58/1
  KeSMSwSeatTrigWaitTimer/1 -> Terminator_60/1
  Ground74/1 -> acsEntryAll4sBwdReq/1
  Ground75/1 -> acsEntryAll4sBwdSoftInt/1
  Ground76/1 -> acsEntryAll4sBwdNotf1ChimeEventStat/1
  Ground77/1 -> acsEntryAll4sBwdReqSig/1
  AcsEntryAll4sBwdAvl/1 -> Terminator_61/1
  RLDoorAjarSwAct/1 -> Terminator_62/1
  RRDoorAjarSwAct/1 -> Terminator_63/1
  KeSMSwSeatSMSSeatMdTrigGapTimer/1 -> Terminator_64/1
  AcsMdExtMdHMI2LRclReq/1 -> Terminator_65/1
  AcsMdExtMdHMI2RRclReq/1 -> Terminator_66/1
  StPassAcsMdExtReq/1 -> Terminator_67/1
  AcsMdExtAvl/1 -> Terminator_68/1
  Ground78/1 -> acsExtMdReq/1
  Ground79/1 -> acsExtMdSrcTp/1
  Ground80/1 -> SwAcsExtLIntCnt/1
  Ground81/1 -> SRSAcsExtIntCnt/1
  Ground82/1 -> acsMdExtNotf1ChimeEventStat/1
  Ground83/1 -> acsExtSoftInt/1
  Ground84/1 -> SwAcsExtRIntCnt/1
  AcsMdEntyHMI2LRclReq/1 -> AcsEntryMdReq/16(HMI2LRclReq)
  AcsMdEntyHMI2RRclReq/1 -> AcsEntryMdReq/17(HMI2RRclReq)
  FamilyMdHMI2RRclReq/1 -> Terminator_11/1
  StPassCmprtMdHMIReqExt2/1 -> [StPassCmprtMdHMIReqExt2]
  [PassCmprtMdHMIReqExt] -> UnfoldMdReq/9(PassCmprtMdHMIReqExt)
  [StPassCmprtMdHMIReqExt2] -> UnfoldMdReq/10(StPassCmprtMdHMIReqExt2)
  Big4SeatMdReq/1(Big4SeatReq) -> Big4SeatReq/1
  Big4SeatMdReq/2(Big4SeatsrcReqTp) -> Big4SeatsrcReqTp/1
  Big4SeatMdReq/3(Big4SeatSoftInt) -> Big4SeatSoftInt/1
  Big4SeatMdReq/4(Big4SeatNotf1ChimeEventStat) -> Big4SeatNotf1ChimeEventStat/1
  [StPassCmprtMdHMIReqExt2] -> Big4SeatMdReq/1(StPassCmprtMdHMIReqExt2)
  StPassUnfold3LReq/1 -> UnfoldMdReq/11(StPassUnfold3LReq)
  UnfoldMdReq/9(Unfold3LSoftInt) -> Unfold3LSoftInt/1
  UnfoldMdReq/10(Unfold3RSoftInt) -> Unfold3RSoftInt/1
  VipMdRtAvl/1 -> [ExVipRMdAvl], [VipMdRtAvl]
  [VipMdRtAvl] -> VipMdReq/16(VipMdRtAvl)
  VipRtOutMdAvl/1 -> [VipRtOutMdAvl], [ExVipROutMdAvl]
  [VipRtOutMdAvl] -> VIPOutMdReq/6(VipRtOutMdAvl)
  [StPassCmprtMdHMIReqExt2] -> "ExVIPMdReq "/1(StPassCmprtMdHMIReqExt2)
  [ExVipRMdAvl] -> "ExVIPMdReq "/2(ExVipRMdAvl)
  [ExVipROutMdAvl] -> "ExVIPMdReq "/3(ExVipROutMdAvl)
  "ExVIPMdReq "/1(ExVIPRReq) -> "ExVIPRReq "/1
  "ExVIPMdReq "/2(ExVIPRsrcReqTp) -> ExVIPRsrcReqTp/1
  "ExVIPMdReq "/3(ExVIPRSoftInt) -> ExVIPRSoftInt/1
  "ExVIPMdReq "/4(ExVIPRNotf1ChimeEventStat) -> ExVIPRNotf1ChimeEventStat/1
  "ExVIPMdReq "/5(ExVIPROutReq) -> ExVIPROutReq/1
  "ExVIPMdReq "/6(ExVIPROutsrcReqTp) -> ExVIPROutsrcReqTp/1
  "ExVIPMdReq "/7(ExVIPROutSoftInt) -> ExVIPROutSoftInt/1
  "ExVIPMdReq "/8(ExVIPROutNotf1ChimeEventStat) -> ExVIPROutNotf1ChimeEventStat/1
  Big4SeatAvl/1 -> Big4SeatMdReq/2(Big4SeatAvl)
  AcsMdEntyAvl/1 -> AcsEntryMdReq/12(AcsMdEntyAvl)
  [StPassCmprtMdHMIReqExt2] -> WholeVehMem/1(StPassCmprtMdHMIReqExt2)
  M61WholeVehMemAvl/1 -> WholeVehMem/2(M61WholeVehMemAvl)
  M62WholeVehMemAvl/1 -> WholeVehMem/3(M62WholeVehMemAvl)
  WholeVehMem/1(WholeVehMem1Req) -> WholeVehMem1Req/1
  WholeVehMem/5(WholeVehMem2Req) -> WholeVehMem2Req/1
  WholeVehMem/4(WholeVehMem1Notf1ChimeEventStat) -> WholeVehMem1Notf1ChimeEventStat/1
  WholeVehMem/2(WholeVehMem1srcReqTp) -> WholeVehMem1srcReqTp/1
  WholeVehMem/3(WholeVehMem1SoftInt) -> WholeVehMem1SoftInt/1
  WholeVehMem/8(WholeVehMem2Notf1ChimeEventStat) -> WholeVehMem2Notf1ChimeEventStat/1
  WholeVehMem/7(WholeVehMem2SoftInt) -> WholeVehMem2SoftInt/1
  WholeVehMem/6(WholeVehMem2srcReqTp) -> WholeVehMem2srcReqTp/1
  StPassCmprtMdCtrl_Md1_VCUConfig/1 -> AcsEntryMdReq/18(StPassCmprtMdCtrl_Md1_VCUConfig)
  StSrv_StMd1_Config/1 -> AcsEntryMdReq/19(StSrv_StMd1_Config)
  StPassCmprtMdCtrl_Md10_VCUConfig/1 -> VipMdReq/21(StPassCmprtMdCtrl_Md10_VCUConfig)
  StPassCmprtMdCtrl_Md12_VCUConfig/1 -> VipMdReq/22(StPassCmprtMdCtrl_Md12_VCUConfig)
  StPassCmprtMdCtrl_Md2_VCUConfig/1 -> VipMdReq/23(StPassCmprtMdCtrl_Md2_VCUConfig)
  StSrv_StMd10_Config/1 -> VipMdReq/24(StSrv_StMd10_Config)
  StSrv_StMd12_Config/1 -> VipMdReq/25(StSrv_StMd12_Config)
  StSrv_StMd2_Config/1 -> VipMdReq/26(StSrv_StMd2_Config)
  StPassCmprtMdCtrl_Md3_VCUConfig/1 -> LugMdReq/21(StPassCmprtMdCtrl_Md3_VCUConfig)
  StPassCmprtMdCtrl_Md8_VCUConfig/1 -> LugMdReq/22(StPassCmprtMdCtrl_Md8_VCUConfig)
  StPassCmprtMdCtrl_Md9_VCUConfig/1 -> LugMdReq/23(StPassCmprtMdCtrl_Md9_VCUConfig)
  StSrv_StMd3_Config/1 -> LugMdReq/24(StSrv_StMd3_Config)
  StSrv_StMd8_Config/1 -> LugMdReq/25(StSrv_StMd8_Config)
  StSrv_StMd9_Config/1 -> LugMdReq/26(StSrv_StMd9_Config)
  StPassCmprtMdCtrl_Md11_VCUConfig/1 -> RecoveryMdReq/18(StPassCmprtMdCtrl_Md11_VCUConfig)
  StPassCmprtMdCtrl_Md13_VCUConfig/1 -> RecoveryMdReq/19(StPassCmprtMdCtrl_Md13_VCUConfig)
  StSrv_StMd11_Config/1 -> RecoveryMdReq/20(StSrv_StMd11_Config)
  StSrv_StMd13_Config/1 -> RecoveryMdReq/21(StSrv_StMd13_Config)
  StPassCmprtMdCtrl_Md30_VCUConfig/1 -> PasReclinerEntryMdReq/7(StPassCmprtMdCtrl_Md30_VCUConfig)
  StPassCmprtMdCtrl_Md27_VCUConfig/1 -> VIPOutMdReq/7(StPassCmprtMdCtrl_Md27_VCUConfig)
  StPassCmprtMdCtrl_Md28_VCUConfig/1 -> VIPOutMdReq/8(StPassCmprtMdCtrl_Md28_VCUConfig)
  StPassCmprtMdCtrl_Md29_VCUConfig/1 -> VIPOutMdReq/9(StPassCmprtMdCtrl_Md29_VCUConfig)
  StSrv_StMd27_Config/1 -> VIPOutMdReq/10(StSrv_StMd27_Config)
  StSrv_StMd28_Config/1 -> VIPOutMdReq/11(StSrv_StMd28_Config)
  StSrv_StMd29_Config/1 -> VIPOutMdReq/12(StSrv_StMd29_Config)
  StSrv_StMd30_Config/1 -> PasReclinerEntryMdReq/8(StSrv_StMd30_Config)
  StPassCmprtMdCtrl_Md31_VCUConfig/1 -> PasReclinerExitMdReq/7(StPassCmprtMdCtrl_Md31_VCUConfig)
  StSrv_StMd31_Config/1 -> PasReclinerExitMdReq/8(StSrv_StMd31_Config)
  StPassCmprtMdCtrl_Md32_VCUConfig/1 -> UnfoldMdReq/12(StPassCmprtMdCtrl_Md32_VCUConfig)
  StPassCmprtMdCtrl_Md53_VCUConfig/1 -> UnfoldMdReq/13(StPassCmprtMdCtrl_Md53_VCUConfig)
  StSrv_StMd32_Config/1 -> UnfoldMdReq/14(StSrv_StMd32_Config)
  StPassCmprtMdCtrl_Md56_VCUConfig/1 -> Big4SeatMdReq/3(StPassCmprtMdCtrl_Md56_VCUConfig)
  StPassCmprtMdCtrl_Md57_VCUConfig/1 -> "ExVIPMdReq "/4(StPassCmprtMdCtrl_Md57_VCUConfig)
  StPassCmprtMdCtrl_Md58_VCUConfig/1 -> "ExVIPMdReq "/5(StPassCmprtMdCtrl_Md58_VCUConfig)
  StPassCmprtMdCtrl_Md61_VCUConfig/1 -> WholeVehMem/4(StPassCmprtMdCtrl_Md61_VCUConfig)
  StPassCmprtMdCtrl_Md62_VCUConfig/1 -> WholeVehMem/5(StPassCmprtMdCtrl_Md62_VCUConfig)

== system ModeInputHandle/ModelInputHandleRunnable_sys/Subsystem1/AcsEntry4s2LMdReq ==
  note: // PassAcsEntry4s2LReq ---》 remote
  EZE4SSwReq : Inport
  AcsEntry4s2LHMI2LRclReq : Inport  Port=2
  PassAcsEntry4s2LReq : Inport  Port=3
  PassCmprtMdHMIReqExt : Inport  Port=4
  SRSSlctSwReq : Inport  Port=5
  SRSCnfmSwReq : Inport  Port=6
  buttonLongPressedThrshhldTm : Inport  Port=7
  curMode : Inport  Port=8
  SRSActiveValidTm : Inport  Port=9
  AcsEntry4s2LAvl : Inport  Port=10
  SRSMode : Inport  Port=11
  AND{,2,4..5} (4 alike) : Logic  AllPortsSameDT=off  OutDataTypeStr=boolean
  ButtonLongPressed2 : Subsystem  AncestorBlock=MSMLib/ButtonLongPressed
  ButtonLongPressed3 : Subsystem  AncestorBlock=MSMLib/ButtonLongPressed
  ConfirmRequireSource : MSMLib/ConfirmRequireSource  SystemSampleTime=-1
  Constant : Constant  Value=MdReqTp1.MdReqTp_Start
  Constant1 : Constant  Value=SRSMode1.SRSSlctSwStat_EzeEntry4s2L  OutDataTypeStr=Enum:SRSMode1
  Constant2 : Constant  Value=CmprtMdHMIReqExtTp1.CmprtMdHMIReqExtTp_Mode21  OutDataTypeStr=Enum:CmprtMdHMIReqExtTp1
  Constant3 : Constant  Value=CmprtMdHMIReqExtTp1.CmprtMdHMIReqExtTp_NoAction  OutDataTypeStr=Enum:CmprtMdHMIReqExtTp1
  Constant4 : Constant  Value=true  OutDataTypeStr=boolean
  Constant5 : Constant  Value=0  OutDataTypeStr=uint8
  Constant8 : Constant  Value=7  OutDataTypeStr=uint8
  Constant9 : Constant  Value=EZESwReq1.EZE_IN  OutDataTypeStr=Enum: EZESwReq1
  Equal{,2,4,6} (4 alike) : RelationalOperator  Operator===  OutDataTypeStr=boolean  RndMeth=Simplest
  Equal1 : RelationalOperator  Operator=~=  OutDataTypeStr=boolean  RndMeth=Simplest
  Equal3 : RelationalOperator  Operator=~=  OutDataTypeStr=boolean  RndMeth=Simplest
  Equal5 : RelationalOperator  Operator=~=  OutDataTypeStr=boolean  RndMeth=Simplest
  Ground2 : Ground
  Logical Operator : Logic  Operator=OR  Inputs=5  AllPortsSameDT=off  OutDataTypeStr=boolean
  NOT : Logic  Operator=NOT  AllPortsSameDT=off  OutDataTypeStr=boolean
  OR1 : Logic  Operator=OR  Inputs=3  AllPortsSameDT=off  OutDataTypeStr=boolean
  Relational Operator3 : RelationalOperator  Operator===  OutDataTypeStr=boolean  RndMeth=Simplest
  SRSReq : MSMLib/SRSReq  SystemSampleTime=-1
  SWIntSrc_S : MSMLib/SWIntSrc_S  SystemSampleTime=-1
  Switch1 : Switch  Criteria=u2 > Threshold
  Switch2 : Switch  Criteria=u2 > Threshold
  Unit Delay : UnitDelay  InitialCondition=e  SampleTime=-1
  Unit Delay1 : UnitDelay  InitialCondition=g  SampleTime=-1
  Unit Delay{2..5} (4 alike) : UnitDelay  SampleTime=-1
  Unit Delay6 : UnitDelay  InitialCondition=d  SampleTime=-1
  acsEntry4s2LReq : Outport  VectorParamsAs1DForOutWhenUnconnected=on
  srcReqTp : Outport  Port=2  VectorParamsAs1DForOutWhenUnconnected=on
  "SwAcsEntry4s2LIntCnt " : Outport  Port=3
  SRSAcsEntry4s2LIntCnt : Outport  Port=4
  Notf1ChimeEventStat : Outport  Port=5
  acsEntry4s2LSoftInt : Outport  Port=6  VectorParamsAs1DForOutWhenUnconnected=on
  wires:
  buttonLongPressedThrshhldTm/1 -> [buttonLongPressedThrshhldTm]
  curMode/1 -> [curMode]
  Constant5/1 -> ButtonLongPressed2/2(longPressThrshhldTm)
  [curMode] -> ButtonLongPressed2/3(curMdState)
  SRSSlctSwReq/1 -> SRSReq/1
  SRSCnfmSwReq/1 -> ButtonLongPressed2/5(SRSCnfmSwReq), SRSReq/3
  Constant1/1 -> SRSReq/4, ButtonLongPressed2/4(CmpReq)
  SRSActiveValidTm/1 -> SRSReq/2
  SRSReq/1 -> ButtonLongPressed2/1(modeReq)
  ButtonLongPressed2/2(mdInterruptCnt) -> SRSAcsEntry4s2LIntCnt/1
  Constant/1 -> Equal1/2, Equal/2
  Unit Delay/1 -> Equal1/1
  Equal/1 -> AND/1
  Equal1/1 -> AND/2
  [SwMdReq] -> Logical Operator/1, ConfirmRequireSource/1
  AND/1 -> [HMI2LReq]
  Constant4/1 -> Equal4/2, Equal5/2
  PassAcsEntry4s2LReq/1 -> Unit Delay2/1, Equal4/1
  Equal4/1 -> AND2/1
  Equal5/1 -> AND2/2
  AND2/1 -> [PassAcsEntry4s2LReq]
  Unit Delay2/1 -> Equal5/1
  [passCmprtMdHMIReq_AcsEntry4s2L] -> Logical Operator/4, OR1/3, ConfirmRequireSource/4
  [SRSReq] -> Logical Operator/5, ConfirmRequireSource/6
  [PassAcsEntry4s2LReq] -> Logical Operator/3, OR1/2, ConfirmRequireSource/5
  Logical Operator/1 -> AND4/1, Switch1/1
  AcsEntry4s2LAvl/1 -> Switch2/2, NOT/1, Switch1/2
  Switch1/1 -> Unit Delay4/1, acsEntry4s2LReq/1
  Unit Delay4/1 -> Switch1/3
  NOT/1 -> AND4/2
  AND4/1 -> Notf1ChimeEventStat/1
  Switch2/1 -> Unit Delay5/1, acsEntry4s2LSoftInt/1
  Unit Delay5/1 -> Switch2/3
  OR1/1 -> Switch2/1
  [HMI2LReq] -> Logical Operator/2, ConfirmRequireSource/2, OR1/1
  ConfirmRequireSource/1 -> srcReqTp/1
  SRSMode/1 -> Unit Delay6/1
  Unit Delay6/1 -> ButtonLongPressed2/6(SRSMode)
  ButtonLongPressed2/1(mdReq) -> [SRSReq]
  AcsEntry4s2LHMI2LRclReq/1 -> Unit Delay/1, Equal/1
  AND5/1 -> [passCmprtMdHMIReq_AcsEntry4s2L]
  Unit Delay1/1 -> Equal2/1
  Constant2/1 -> Relational Operator3/2
  PassCmprtMdHMIReqExt/1 -> Unit Delay1/1, Relational Operator3/1
  Relational Operator3/1 -> AND5/1
  Constant3/1 -> Equal2/2
  Equal2/1 -> AND5/2
  [buttonLongPressedThrshhldTm] -> ButtonLongPressed3/2(longPressThrshhldTm)
  ButtonLongPressed3/1(mdReq) -> [SwMdReq]
  Unit Delay3/1 -> Equal3/2
  Constant8/1 -> SWIntSrc_S/2
  Equal3/1 -> SWIntSrc_S/1
  ButtonLongPressed3/2(mdInterruptCnt) -> "SwAcsEntry4s2LIntCnt "/1, Unit Delay3/1, Equal3/1
  Ground2/1 -> ConfirmRequireSource/3
  EZE4SSwReq/1 -> Equal6/1
  Constant9/1 -> Equal6/2
  Equal6/1 -> ButtonLongPressed3/1(modeReq)
